simulink model "cl_Nested"  (R2024b)
settings: Solver=VariableStepAuto  StartTime=0.0  StopTime=Tmax  RelTol=1e-3
values from neighbouring files (symbols this model uses):
  Gear = [25 20 25]    [controlled_robot_def_Nested.m]    (also in controlled_robot_def_PD.m; controlled_robot_def_PID.m; controlled_robot_def_ctorque.m; controlled_robot_def_freedfwrd.m)
  Ki = [0.06 0.06 0.06]    [controlled_robot_def_Nested.m]
  km = [10 10 10]    [controlled_robot_def_Nested.m]    (also in controlled_robot_def_PD.m; controlled_robot_def_PID.m; controlled_robot_def_ctorque.m; controlled_robot_def_freedfwrd.m)
  Kp = [50 50 50]    [controlled_robot_def_Nested.m]    (also in controlled_robot_def_ctorque.m = 20; controlled_robot_def_freedfwrd.m = [100])
  Kv = [3.5 3.5 3.5]    [controlled_robot_def_Nested.m]
  q_inicial = [0 0 0]    [circle_drawing.m]    (also in controlled_robot_def_Nested.m; controlled_robot_def_PD.m; controlled_robot_def_PID.m; controlled_robot_def_ctorque.m)
  qf = [pi/2 pi/8 pi/8]    [controlled_robot_def_Nested.m]    (also in controlled_robot_def_PD.m; controlled_robot_def_PID.m; controlled_robot_def_ctorque.m; controlled_robot_def_freedfwrd.m)
  robot_3dof = SerialLink(L, 'name', 'Robot 3-DOF')    [circle_drawing.m]    (also in controlled_robot_def_Nested.m; controlled_robot_def_PD.m; controlled_robot_def_PID.m; controlled_robot_def_ctorque.m)
  Tm = Ts_calculated    [controlled_robot_def_Nested.m]    (also in controlled_robot_def_PD.m; controlled_robot_def_PID.m; controlled_robot_def_ctorque.m; controlled_robot_def_freedfwrd.m)
  unc = 0.2    [controlled_robot_def_Nested.m]    (also in controlled_robot_def_PD.m; controlled_robot_def_PID.m = 0; controlled_robot_def_ctorque.m; controlled_robot_def_freedfwrd.m)
libraries: roblocks x4
settings Model: Creator=pcarn  LastModifiedBy=pablo

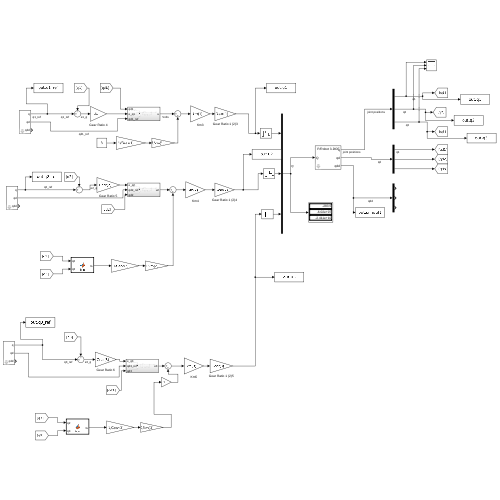
[thumbnail: Simulink's stored preview of the top-level diagram]
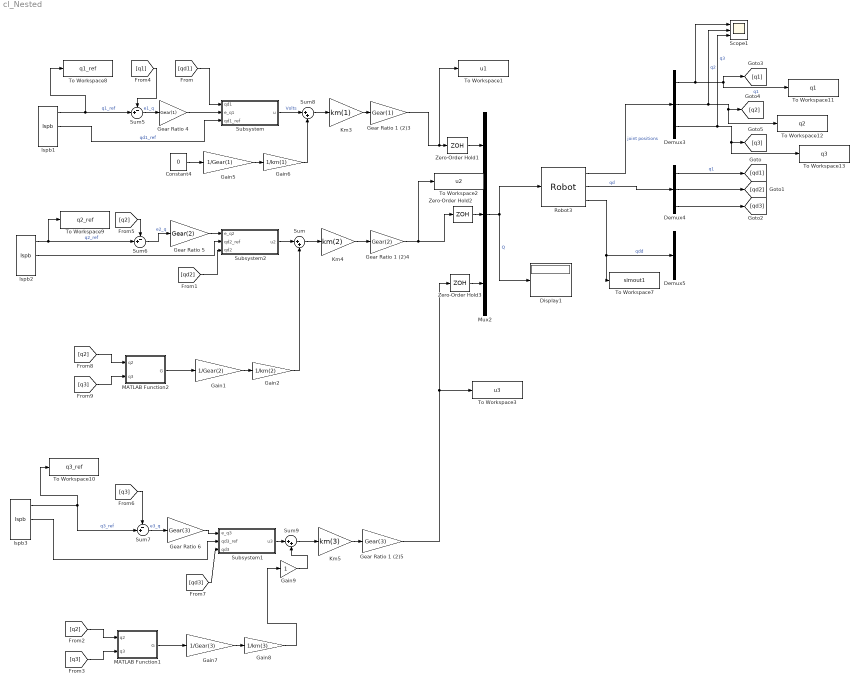
== system cl_Nested ==
  Constant4 : Constant  Value=0
  Demux3 : Demux  Outputs=3
  Demux4 : Demux  Outputs=3
  Demux5 : Demux  Outputs=3
  Display1 : Display
  Gain1 : Gain  Gain=1/Gear(2)
  Gain2 : Gain  Gain=1/km(2)
  Gain5 : Gain  Gain=1/Gear(1)
  Gain6 : Gain  Gain=1/km(1)
  Gain7 : Gain  Gain=1/Gear(3)
  Gain8 : Gain  Gain=1/km(3)
  Gain9 : Gain
  Gear Ratio 1 (2)3 : Gain  Gain=Gear(1)
  Gear Ratio 1 (2)4 : Gain  Gain=Gear(2)
  Gear Ratio 1 (2)5 : Gain  Gain=Gear(3)
  Gear Ratio 4 : Gain  Gain=Gear(1)
  Gear Ratio 5 : Gain  Gain=Gear(2)
  Gear Ratio 6 : Gain  Gain=Gear(3)
  Km3 : Gain  Gain=km(1)
  Km4 : Gain  Gain=km(2)
  Km5 : Gain  Gain=km(3)
  MATLAB Function1 : MATLAB Function  TreatAsAtomicUnit=on
  MATLAB Function2 : MATLAB Function  TreatAsAtomicUnit=on
  Mux2 : Mux  Inputs=3
  Robot3 : roblocks/Arm/Robot  robot=robot_3dof.perturb(unc)  q0=q_inicial
  Scope1 : Scope  NumInputPorts=3
  Subsystem : Subsystem
  Subsystem1 : Subsystem
  Subsystem2 : Subsystem
  Sum : Sum  Inputs=|++
  Sum5 : Sum  Inputs=-+|
  Sum6 : Sum  Inputs=-+|
  Sum7 : Sum  Inputs=-+|
  Sum8 : Sum  Inputs=|++
  Sum9 : Sum  Inputs=|++
  To Workspace1 : ToWorkspace  VariableName=u1  SaveFormat=Timeseries  SampleTime=-1
  To Workspace10 : ToWorkspace  VariableName=q3_ref  SaveFormat=Timeseries  SampleTime=-1
  To Workspace11 : ToWorkspace  VariableName=q1  SaveFormat=Timeseries  SampleTime=-1
  To Workspace12 : ToWorkspace  VariableName=q2  SaveFormat=Timeseries  SampleTime=-1
  To Workspace13 : ToWorkspace  VariableName=q3  SaveFormat=Timeseries  SampleTime=-1
  To Workspace2 : ToWorkspace  VariableName=u2  SaveFormat=Timeseries  SampleTime=-1
  To Workspace3 : ToWorkspace  VariableName=u3  SaveFormat=Timeseries  SampleTime=-1
  To Workspace7 : ToWorkspace  VariableName=simout1  SaveFormat=Timeseries  SampleTime=-1
  To Workspace8 : ToWorkspace  VariableName=q1_ref  SaveFormat=Timeseries  SampleTime=-1
  To Workspace9 : ToWorkspace  VariableName=q2_ref  SaveFormat=Timeseries  SampleTime=-1
  Zero-Order Hold1 : ZeroOrderHold  SampleTime=Tm
  Zero-Order Hold2 : ZeroOrderHold  SampleTime=Tm
  Zero-Order Hold3 : ZeroOrderHold  SampleTime=Tm
  lspb1 : roblocks/Toolbox/lspb  q0=q_inicial(1)  qf=qf(1)  tmax=Tmax
  lspb2 : roblocks/Toolbox/lspb  q0=q_inicial(2)  qf=qf(2)  tmax=Tmax
  lspb3 : roblocks/Toolbox/lspb  q0=q_inicial(3)  qf=qf(3)  tmax=Tmax
  wires:
  Gain6/1 -> Sum8/2
  Gear Ratio 5/1 -> Subsystem2/1(e_q2)
  Sum9/1 -> Km5/1
  Subsystem1/1(u3) -> Sum9/1
  Gear Ratio 1 (2)3/1 -> To Workspace1/1, Zero-Order Hold1/1
  Km5/1 -> Gear Ratio 1 (2)5/1
  Robot3/3 -> Demux5/1, To Workspace7/1  "qdd"
  lspb1/1 -> To Workspace8/1, Sum5/2  "q1_ref"
  Gear Ratio 1 (2)5/1 -> Zero-Order Hold3/1, To Workspace3/1
  Sum8/1 -> Km3/1
  Km3/1 -> Gear Ratio 1 (2)3/1
  MATLAB Function1/1(G) -> Gain7/1
  Demux3/2 -> Scope1/2, To Workspace12/1, [q2]  "q2"
  Demux3/1 -> Scope1/1, [q1], To Workspace11/1  "q1"
  Sum5/1 -> Gear Ratio 4/1  "e1_q"
  Gain7/1 -> Gain8/1
  Mux2/1 -> Display1/1, Robot3/1  "Q"
  Constant4/1 -> Gain5/1
  Demux3/3 -> Scope1/3, To Workspace13/1, [q3]  "q3"
  Sum6/1 -> Gear Ratio 5/1  "e2_q"
  Gain8/1 -> Gain9/1
  lspb3/1 -> To Workspace10/1, Sum7/2  "q3_ref"
  Robot3/1 -> Demux3/1  "joint positions"
  Gain5/1 -> Gain6/1
  Subsystem/1(u) -> Sum8/1  "Volts"
  Gear Ratio 6/1 -> Subsystem1/1(e_q3)
  Sum7/1 -> Gear Ratio 6/1  "e3_q"
  Km4/1 -> Gear Ratio 1 (2)4/1
  Robot3/2 -> Demux4/1  "qd"
  Gain9/1 -> Sum9/2
  Gear Ratio 1 (2)4/1 -> To Workspace2/1, Zero-Order Hold2/1
  lspb2/1 -> Sum6/2, To Workspace9/1  "q2_ref"
  Gear Ratio 4/1 -> Subsystem/2(e_q1)
  Demux4/1 -> [qd1]  "q1"
  Demux4/2 -> [qd2]
  Demux4/3 -> [qd3]
  [qd1] -> Subsystem/1(qd1)
  lspb1/2 -> Subsystem/3(qd1_ref)  "qd1_ref"
  [qd2] -> Subsystem2/3(qd2)
  lspb2/2 -> Subsystem2/2(qd2_ref)
  [q2] -> MATLAB Function1/1(q2)
  [q3] -> MATLAB Function1/2(q3)
  [q1] -> Sum5/1
  [q2] -> Sum6/1
  [q3] -> Sum7/1
  [qd3] -> Subsystem1/3(qd3)
  lspb3/2 -> Subsystem1/2(qd3_ref)
  Zero-Order Hold1/1 -> Mux2/1
  Zero-Order Hold2/1 -> Mux2/2
  Zero-Order Hold3/1 -> Mux2/3
  [q3] -> MATLAB Function2/2(q3)
  [q2] -> MATLAB Function2/1(q2)
  Gain2/1 -> Sum/2
  Gain1/1 -> Gain2/1
  MATLAB Function2/1(G) -> Gain1/1
  Subsystem2/1(u2) -> Sum/1
  Sum/1 -> Km4/1

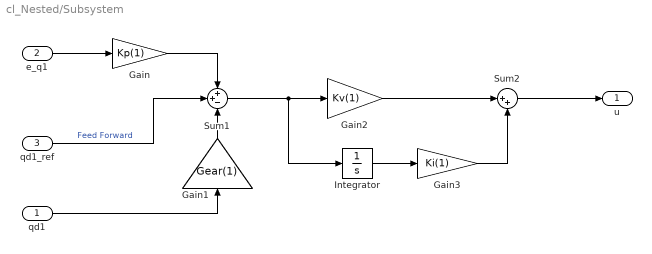
== system cl_Nested/Subsystem ==
  qd1 : Inport
  e_q1 : Inport  Port=2
  qd1_ref : Inport  Port=3
  Gain : Gain  Gain=Kp(1)
  Gain1 : Gain  Gain=Gear(1)
  Gain2 : Gain  Gain=Kv(1)
  Gain3 : Gain  Gain=Ki(1)
  Integrator : Integrator
  Sum1 : Sum  Inputs=++-
  Sum2 : Sum  Inputs=|++
  u : Outport
  wires:
  e_q1/1 -> Gain/1
  Gain/1 -> Sum1/1
  qd1_ref/1 -> Sum1/2  "Feed Forward"
  Sum1/1 -> Integrator/1, Gain2/1
  qd1/1 -> Gain1/1
  Gain1/1 -> Sum1/3
  Integrator/1 -> Gain3/1
  Gain2/1 -> Sum2/1
  Gain3/1 -> Sum2/2
  Sum2/1 -> u/1

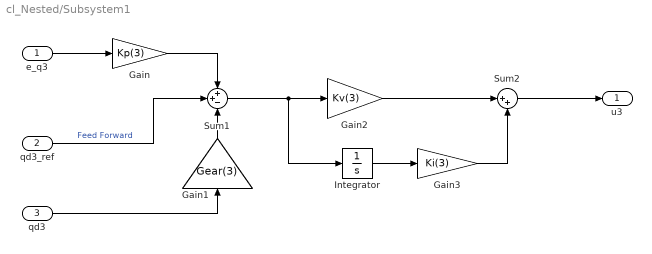
== system cl_Nested/Subsystem1 ==
  e_q3 : Inport
  qd3_ref : Inport  Port=2
  qd3 : Inport  Port=3
  Gain : Gain  Gain=Kp(3)
  Gain1 : Gain  Gain=Gear(3)
  Gain2 : Gain  Gain=Kv(3)
  Gain3 : Gain  Gain=Ki(3)
  Integrator : Integrator
  Sum1 : Sum  Inputs=++-
  Sum2 : Sum  Inputs=|++
  u3 : Outport
  wires:
  e_q3/1 -> Gain/1
  Gain/1 -> Sum1/1
  qd3_ref/1 -> Sum1/2  "Feed Forward"
  Sum1/1 -> Integrator/1, Gain2/1
  qd3/1 -> Gain1/1
  Gain1/1 -> Sum1/3
  Integrator/1 -> Gain3/1
  Gain2/1 -> Sum2/1
  Gain3/1 -> Sum2/2
  Sum2/1 -> u3/1

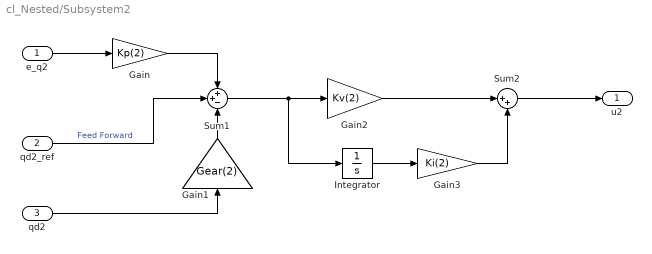
== system cl_Nested/Subsystem2 ==
  e_q2 : Inport
  qd2_ref : Inport  Port=2
  qd2 : Inport  Port=3
  Gain : Gain  Gain=Kp(2)
  Gain1 : Gain  Gain=Gear(2)
  Gain2 : Gain  Gain=Kv(2)
  Gain3 : Gain  Gain=Ki(2)
  Integrator : Integrator
  Sum1 : Sum  Inputs=++-
  Sum2 : Sum  Inputs=|++
  u2 : Outport
  wires:
  Sum2/1 -> u2/1
  Gain3/1 -> Sum2/2
  Gain2/1 -> Sum2/1
  Integrator/1 -> Gain3/1
  Gain1/1 -> Sum1/3
  qd2/1 -> Gain1/1
  Sum1/1 -> Gain2/1, Integrator/1
  qd2_ref/1 -> Sum1/2  "Feed Forward"
  Gain/1 -> Sum1/1
  e_q2/1 -> Gain/1

== matlab function cl_Nested/MATLAB Function2 ==
  data: q2 input; G output; q3 input
function G = fcn(q2, q3)
    
    D = [2 9 5 5 5 5 5 8];

    l1a = 0.9 - 0.04*D(2); 
    l2a = 0.4 + 0.02*D(6); 
    l3a = 0.4 + 0.01*D(3); 
    l4a = 0.5 - 0.02*D(7);
    
    m1 = 4;
    m2 = 2.7;
    m3 = 2;

    g = 9.81;

    
G = g*m3*(l4a*cos(q2 + q3) + l3a*cos(q2) - l2a*sin(q2)) + g*m2*cos(q2 + atan(l2a/l3a))*(l2a^2 + l3a^2)^(1/2);

== matlab function cl_Nested/MATLAB Function1 ==
  data: q2 input; G output; q3 input
function G = fcn(q2, q3)
    
    D = [2 9 5 5 5 5 5 8];

    L1a_val = 0.9 - 0.04*D(2); 
    L2a_val = 0.4 + 0.02*D(6); 
    L3a_val = 0.4 + 0.01*D(3); 
    L4a_val = 0.5 - 0.02*D(7);
    
    m1_val = 4;
    m2_val = 2.7;
    m3_val = 2;

    
G = 9.81*L4a_val*m3_val*cos(q2+q3);
